simulink model "sl_subsys_trigerr1"  (Simulink 7.6)
settings: Solver=ode45  StartTime=0.0  StopTime=10.0  RelTol=1e-3
Description:
  | Example of modeling error - ambiguous execution order due to nonlatched triggered subsystem
settings Model: Creator=The MathWorks Inc.  CovMetricSettings=d  ExtModeAutoUpdateStatusClock=off
settings OptimizationCC: BlockReduction=off  BooleanDataType=off  InitFltsAndDblsToZero=on
settings DebuggingCC: SaveWithParameterizedLinksMsg=none  SignalResolutionControl=TryResolveAllWithWarning  SolverPrmCheckMsg=none  MultiTaskDSMMsg=warning  MultiTaskCondExecSysMsg=none
settings HardwareCC: TargetUnknown=on
settings RTWCC: IncludeERTFirstTime=on
settings CodeAppCC: CustomSymbolStrFcn=$F$N$M
settings GRTTargetCC: TargetFcnLib=ansi_tfl_tmw.mat

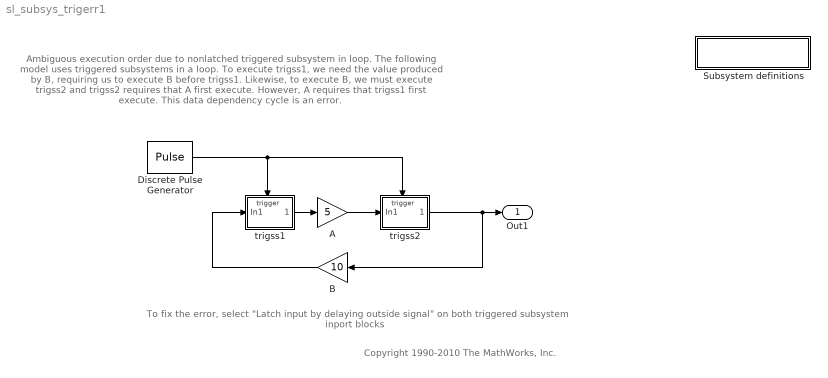
== system sl_subsys_trigerr1 ==
  note: Ambiguous execution order due to nonlatched triggered subsystem in loop.
      |
      | The following model uses triggered subsystems in a loop. To execute
      | trigss1, we need the value produced by B, requiring us to execute
      | B before trigss1. Likewise, to execute B, we must execute trigss2
      | and trigss2 requires that A first execute. However, A requires that
      | trigss1 first execute. This data dependency cycle is an error.
  note: To fix the error, select "Latch input by delaying outside signal"
      | on both triggered subsystem inport blocks
  note: Copyright 1990-2010 The MathWorks, Inc.
  " Subsystem definitions" : Subsystem
      settings: OpenFcn=helpview([matlabroot,'/toolbox/simulink/simdemos/simfeatures/html/sl_subsys_definitions.html']);
      mask Display: disp('Subsystem\ndefinitions')
  A : Gain  Gain=5  SaturateOnIntegerOverflow=on  OutDataTypeStr=Inherit: Same as input  ParamDataTypeStr=Inherit: Same as input
  B : Gain  Gain=10  SaturateOnIntegerOverflow=on  OutDataTypeStr=Inherit: Same as input  ParamDataTypeStr=Inherit: Same as input
  Discrete Pulse Generator : DiscretePulseGenerator
  trigss1 : Subsystem  TreatAsAtomicUnit=on
  trigss2 : Subsystem  TreatAsAtomicUnit=on
  Out1 : Outport
  wires:
  trigss1/1(Out1) -> A/1
  A/1 -> trigss2/1(In1)
  trigss2/1(Out1) -> B/1, Out1/1
  B/1 -> trigss1/1(In1)
  Discrete Pulse Generator/1 -> trigss1/Trigger, trigss2/Trigger

== system sl_subsys_trigerr1/ Subsystem definitions ==

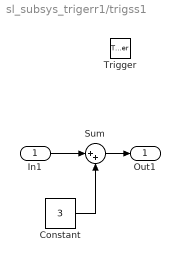
== system sl_subsys_trigerr1/trigss1 ==
  In1 : Inport
  Trigger : TriggerPort
  Constant : Constant  Value=3
  Sum : Sum  Inputs=|++  SaturateOnIntegerOverflow=on  InputSameDT=on  OutDataTypeStr=Inherit: Same as first input
  Out1 : Outport
  wires:
  In1/1 -> Sum/1
  Sum/1 -> Out1/1
  Constant/1 -> Sum/2

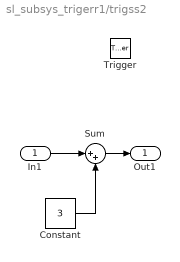
== system sl_subsys_trigerr1/trigss2 ==
  In1 : Inport
  Trigger : TriggerPort
  Constant : Constant  Value=3
  Sum : Sum  Inputs=|++  SaturateOnIntegerOverflow=on  InputSameDT=on  OutDataTypeStr=Inherit: Same as first input
  Out1 : Outport
  wires:
  Constant/1 -> Sum/2
  Sum/1 -> Out1/1
  In1/1 -> Sum/1
